simulink model "AGI_hydrogen"  (R2024b)
settings: Solver=VariableStepAuto  StartTime=0.0  StopTime=3  RelTol=1e-3
values from neighbouring files (symbols this model uses):
  ControlSampleTime = 1/8000    (= 0.000125)    [initTPHardware.m]
  HWSampleTime = ControlSampleTime/4    (= 3.125e-05)    [initTPHardware.m]
undefined symbols (not defined in the file or in its folder): DiscIntNeverNeededParam, fault_dur, Grid, Ion, LCL, Lithium, Manage, Param, SM, t_fault, Ts_Control, Ts_Power, V_DC, VSMCTRL
libraries: FriedrichLibrary x19, simulink x8, spsSeriesRLCBranchLib x7, spsThreePhaseSeriesRLCBranchLib x6, TriphaseHardwaremodule x6, powerlib_extras x6, spsThreePhaseVIMeasurementLib x5, spsVoltageMeasurementLib x5, spsThreePhaseBreakerLib x4, slpidlib x4, spsUniversalBridgeLib x3, spsCurrentMeasurementLib x3
(part 3 of 4)

== system AGI_hydrogen/Battery/VSM1/VSM/CONTROL/Virtual Circuit mit R und L ==
  Param : Inport
  Reset : Inport  Port=2
  i_dq0 : Inport  Port=3
  Phi : Inport  Port=4
  Bus Selector : BusSelector  OutputSignals=R1,L1
  Bus Selector1 : BusSelector  OutputSignals=R1t,tauR,L1t,tauL
  Current Predictor : Subsystem  Commented=on
  L_Matrix : Gain  Gain=[0 -1 0;1 0 0; 0 0 0]
  L_Matrix1 : Gain  Gain=[0 -1 0;1 0 0; 0 0 0]
  PT1 : Subsystem  mask{K=1, Init=0, Ts=ControlSampleTime}
      mask prompts: K "Gain"; Init "Initial input"; Ts "Sample time"
      mask DialogControl DescGroupVar Prompt: PT1 discrete
      mask DialogControl DescTextVar Prompt: Simple discrete PT1
      mask Display:
      | text(0.5,0.5,get_param(gcb,'K'),'HorizontalAlignment','center','VerticalAlignment','Bottom')
      | text(0.5,0.5,'1 + s.tau','HorizontalAlignment','center','VerticalAlignment','Top')
      | plot([0.3 0.7],[0.5 0.5])
  PT2 : Subsystem  mask{K=1, Init=0, Ts=ControlSampleTime}
      mask prompts: K "Gain"; Init "Initial input"; Ts "Sample time"
      mask DialogControl DescGroupVar Prompt: PT1 discrete
      mask DialogControl DescTextVar Prompt: Simple discrete PT1
      mask Display:
      | text(0.5,0.5,get_param(gcb,'K'),'HorizontalAlignment','center','VerticalAlignment','Bottom')
      | text(0.5,0.5,'1 + s.tau','HorizontalAlignment','center','VerticalAlignment','Top')
      | plot([0.3 0.7],[0.5 0.5])
  "Param " : InportShadow
  Phi1 : InportShadow  Port=4
  Product : Product  Multiplication=Matrix(*)
  Product1 : Product  Multiplication=Matrix(*)
  Product2 : Product  Multiplication=Matrix(*)
  R_Matrix : Gain  Gain=[1 0 0;0 1 0; 0 0 0]
  R_Matrix1 : Gain  Gain=[1 0 0;0 1 0; 0 0 0]
  Reset1 : InportShadow  Port=2
  Sum : Sum  Inputs=++|
  Sum1 : Sum  Inputs=++|
  Sum2 : Sum  Inputs=|++
  " u_dq0" : Outport
  wires:
  Param/1 -> Bus Selector/1
  Bus Selector/1 -> R_Matrix/1  "<R1>"
  i_dq0/1 -> Product/2, PT2/1(U), PT1/1(U)
  Bus Selector/2 -> L_Matrix/1  "<L1>"
  L_Matrix/1 -> Sum/1
  R_Matrix/1 -> Sum/2
  Sum/1 -> Product/1
  "Param "/1 -> Bus Selector1/1
  R_Matrix1/1 -> Product1/1
  Product1/1 -> Sum1/1
  Bus Selector1/1 -> R_Matrix1/1  "<R1t>"
  Bus Selector1/4 -> PT2/2(tau)  "<tauL>"
  Bus Selector1/2 -> PT1/2(tau)  "<tauR>"
  Bus Selector1/3 -> L_Matrix1/1  "<L1t>"
  L_Matrix1/1 -> Product2/1
  Product2/1 -> Sum1/2
  Sum2/1 -> " u_dq0"/1
  PT1/1(Y) -> Product1/2
  Phi/1 -> PT1/4(Phi)
  Phi1/1 -> PT2/4(Phi)
  Reset/1 -> PT1/3(Reset)
  Reset1/1 -> PT2/3(Reset)
  PT2/1(Y) -> Product2/2
  Product/1 -> Sum2/1

== system AGI_hydrogen/Battery/VSM1/VSM/CONTROL/Virtual Circuit1 ==
  Param : Inport
  Reset : Inport  Port=2
  i_dq0 : Inport  Port=3
  Phi : Inport  Port=4
  Bus Selector : BusSelector  OutputSignals=R1,L1
  Bus Selector1 : BusSelector  OutputSignals=R1t,tauR,L1t,tauL
  Current Predictor : Subsystem  Commented=on
  L_Matrix : Gain  Gain=[0 -1 0;1 0 0; 0 0 0]
  L_Matrix1 : Gain  Gain=[0 -1 0;1 0 0; 0 0 0]
  PT1 : Subsystem  mask{K=1, Init=0, Ts=ControlSampleTime}
      mask prompts: K "Gain"; Init "Initial input"; Ts "Sample time"
      mask DialogControl DescGroupVar Prompt: PT1 discrete
      mask DialogControl DescTextVar Prompt: Simple discrete PT1
      mask Display:
      | text(0.5,0.5,get_param(gcb,'K'),'HorizontalAlignment','center','VerticalAlignment','Bottom')
      | text(0.5,0.5,'1 + s.tau','HorizontalAlignment','center','VerticalAlignment','Top')
      | plot([0.3 0.7],[0.5 0.5])
  PT2 : Subsystem  Commented=on  mask{K=1, Init=0, Ts=ControlSampleTime}
      mask prompts: K "Gain"; Init "Initial input"; Ts "Sample time"
      mask DialogControl DescGroupVar Prompt: PT1 discrete
      mask DialogControl DescTextVar Prompt: Simple discrete PT1
      mask Display:
      | text(0.5,0.5,get_param(gcb,'K'),'HorizontalAlignment','center','VerticalAlignment','Bottom')
      | text(0.5,0.5,'1 + s.tau','HorizontalAlignment','center','VerticalAlignment','Top')
      | plot([0.3 0.7],[0.5 0.5])
  "Param " : InportShadow
  Phi1 : InportShadow  Port=4
  Product : Product  Multiplication=Matrix(*)
  Product1 : Product  Multiplication=Matrix(*)
  Product2 : Product  Commented=on  Multiplication=Matrix(*)
  Product3 : Product  Multiplication=Matrix(*)
  R_Matrix : Gain  Gain=[1 0 0;0 1 0; 0 0 0]
  R_Matrix1 : Gain  Gain=[1 0 0;0 1 0; 0 0 0]
  Reset1 : InportShadow  Port=2
  Scope : Scope  NumInputPorts=2
  Scope1 : Scope
  Sum : Sum  Inputs=++|
  Sum1 : Sum  Inputs=++|
  Sum2 : Sum  Inputs=|++
  " u_dq0" : Outport
  wires:
  Param/1 -> Bus Selector/1
  Bus Selector/1 -> R_Matrix/1  "<R1>"
  i_dq0/1 -> PT2/1(U), PT1/1(U), Product3/2, Product/2
  Bus Selector/2 -> L_Matrix/1  "<L1>"
  L_Matrix/1 -> Sum/1
  R_Matrix/1 -> Product3/1, Sum/2
  Sum/1 -> Product/1
  "Param "/1 -> Bus Selector1/1
  Product/1 -> Sum2/1
  R_Matrix1/1 -> Product1/1
  Product1/1 -> Scope/2, Sum1/1
  Bus Selector1/1 -> R_Matrix1/1  "<R1t>"
  Bus Selector1/4 -> PT2/2(tau)  "<tauL>"
  Bus Selector1/2 -> PT1/2(tau)  "<tauR>"
  Bus Selector1/3 -> L_Matrix1/1  "<L1t>"
  L_Matrix1/1 -> Product2/1
  PT2/1(Y) -> Product2/2
  Product2/1 -> Scope1/1, Sum1/2
  Sum1/1 -> Sum2/2
  Sum2/1 -> " u_dq0"/1
  PT1/1(Y) -> Product1/2
  Phi1/1 -> PT2/4(Phi)
  Reset/1 -> PT1/3(Reset)
  Reset1/1 -> PT2/3(Reset)
  Product3/1 -> Scope/1

== system AGI_hydrogen/Battery/VSM1/VSM/CONTROL/active_damping ==
  enable_damp_dq : Inport
  Reset : Inport  Port=2
  u_dq0 : Inport  Port=3
  Phi : Inport  Port=4
  Bus Selector : BusSelector  OutputSignals=Damp_dq,Damp_dq,Damp_CM,OmLead,OmLag
  Integrator (inertia) : DiscreteIntegrator  gainval=1  ExternalReset=rising  InitialConditionSource=external  InitialCondition=1  SampleTime=ControlSampleTime  ICPrevOutput=DiscIntNeverNeededParam  ICPrevScaledInput=DiscIntNeverNeededParam
  Mux : Mux  Inputs=3
  Product{,1..3} (4 alike) : Product
  Sum : Sum  Inputs=|+-
  Sum2 : Sum  Inputs=++|
  Unit Delay2 : UnitDelay  InitialCondition=[0 0 0]  SampleTime=ControlSampleTime  HasFrameUpgradeWarning=on
  dq0->ab0 phi : FriedrichLibrary/Transformations/dq0->ab0 phi  SystemSampleTime=-1  VariantActivationTime=update diagram  AllowFlexibleInterface=on  Latency=0  AutoFrameSizeCalculation=off
  damp_dq0 : Outport  VectorParamsAs1DForOutWhenUnconnected=off
  wires:
  Product2/1 -> Sum/1
  Integrator (inertia)/1 -> Unit Delay2/1, Sum2/2
  Product3/1 -> Sum/2
  Sum2/1 -> Product3/1, Product1/2
  Sum/1 -> Integrator (inertia)/1
  enable_damp_dq/1 -> Bus Selector/1
  Bus Selector/1 -> Mux/1  "<Damp_dq>"
  Bus Selector/2 -> Mux/2  "<Damp_dq>"
  Bus Selector/3 -> Mux/3  "<Damp_CM>"
  u_dq0/1 -> Product/2
  Product/1 -> Sum2/1, Product2/2
  Mux/1 -> Product1/1, Product/1  "enable"
  Product1/1 -> damp_dq0/1
  Phi/1 -> dq0->ab0 phi/2
  Reset/1 -> Integrator (inertia)/2
  Unit Delay2/1 -> dq0->ab0 phi/1
  dq0->ab0 phi/1 -> Integrator (inertia)/3
  Bus Selector/4 -> Product2/1  "<OmLead>"
  Bus Selector/5 -> Product3/2  "<OmLag>"

== system AGI_hydrogen/Battery/VSM1/VSM/CONTROL/dq0 to duty ==
  phi_rad : Inport
  u_dq0 : Inport  Port=2
  u_dc : Inport  Port=3
  Bias : Bias  Bias=Ctrl.PWM.tauT*Ctrl.PU.omegab  SaturateOnIntegerOverflow=off
  Bus Creator3 : BusCreator  Inputs=2
  Divide : Product  Inputs=*/
  Gain : Gain  Gain=eye(NrChannels,3)  Multiplication=Matrix(K*u)
  Modulation : FriedrichLibrary/Transformations/Modulation  Method=Sine Modulation  Ts=ControlSampleTime
  SMA : FriedrichLibrary/Discrete Stuff/SMA  n_samples=1/ControlSampleTime/100  init_out=0
  Saturation : Saturate  UpperLimit=inf  LowerLimit=1
  Signal Specification1 : SignalSpecification
  dq0->ab0 phi : FriedrichLibrary/Transformations/dq0->ab0 phi  SystemSampleTime=-1  VariantActivationTime=update diagram  AllowFlexibleInterface=on  Latency=0  AutoFrameSizeCalculation=off
  d : Outport  VectorParamsAs1DForOutWhenUnconnected=off
  pwmDiag : Outport  Port=2  VectorParamsAs1DForOutWhenUnconnected=off
  wires:
  phi_rad/1 -> Bus Creator3/2, Bias/1  "phi"
  u_dq0/1 -> dq0->ab0 phi/1
  Divide/1 -> Modulation/1  "ab0 norm"
  dq0->ab0 phi/1 -> Divide/1
  Modulation/1 -> Gain/1
  Bias/1 -> dq0->ab0 phi/2
  u_dc/1 -> Saturation/1
  Bus Creator3/1 -> pwmDiag/1  "pwmDiag"
  Gain/1 -> Bus Creator3/1, Signal Specification1/1  "pwm"
  Signal Specification1/1 -> d/1
  Saturation/1 -> SMA/1
  SMA/1 -> Divide/2

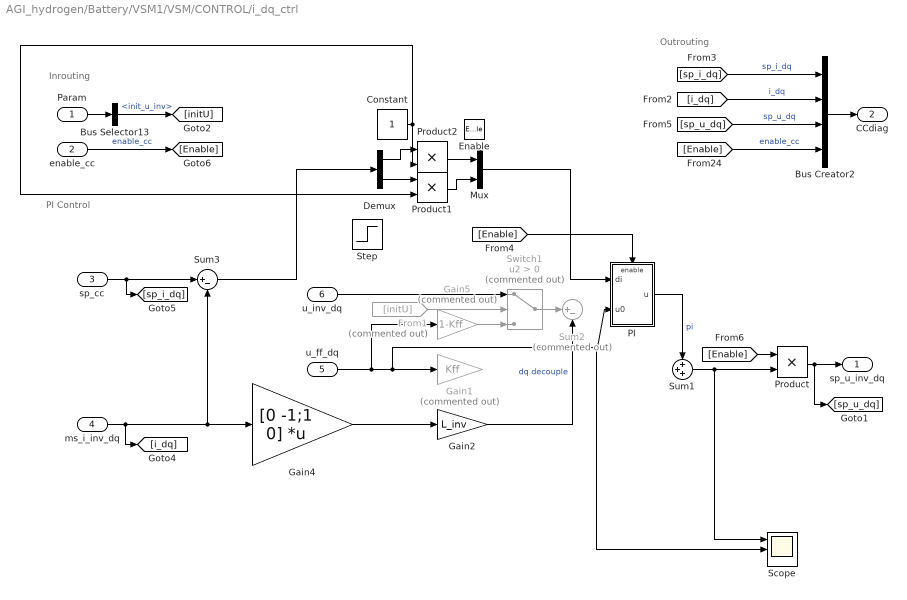
== system AGI_hydrogen/Battery/VSM1/VSM/CONTROL/i_dq_ctrl ==
  note: Inrouting
  note: Outrouting
  note: PI Control
  Param : Inport
  enable_cc : Inport  Port=2
  sp_cc : Inport  Port=3
  ms_i_inv_dq : Inport  Port=4
  u_ff_dq : Inport  Port=5
  u_inv_dq : Inport  Port=6
  Enable : EnablePort  StatesWhenEnabling=reset
  Bus Creator2 : BusCreator  Inputs=4
  Bus Selector13 : BusSelector  OutputSignals=init_u_inv
  Constant : Constant
  Demux : Demux  Outputs=2
  From1 : From  Commented=on  GotoTag=initU
  Gain1 : Gain  Commented=on  Gain=Kff
  Gain2 : Gain  Gain=L_inv
  Gain4 : Gain  Gain=[0 -1;1 0]  Multiplication=Matrix(K*u)
  Gain5 : Gain  Commented=on  Gain=1-Kff
  Mux : Mux  Inputs=2
  PI : Subsystem
  Product : Product
  Product1 : Product
  Product2 : Product
  Scope : Scope  NumInputPorts=3
  Step : Step  Time=8  Before=1  After=0  SampleTime=0
  Sum1 : Sum  Inputs=+++
  Sum2 : Sum  Commented=on  Inputs=|+-
  Sum3 : Sum  Inputs=|+-
  Switch1 : Switch  Commented=on  Criteria=u2 > Threshold  SaturateOnIntegerOverflow=off  InputSameDT=off
  sp_u_inv_dq : Outport  VectorParamsAs1DForOutWhenUnconnected=off
  CCdiag : Outport  Port=2  VectorParamsAs1DForOutWhenUnconnected=off
  wires:
  Switch1/1 -> Sum2/1
  Gain4/1 -> Gain2/1
  Gain2/1 -> Sum2/2  "dq decouple"
  From1/1 -> Switch1/2
  Sum1/1 -> Scope/1, Product/2
  u_inv_dq/1 -> Switch1/1
  [Enable] -> PI/Enable
  Sum3/1 -> Demux/1
  sp_cc/1 -> [sp_i_dq], Sum3/1
  Param/1 -> Bus Selector13/1
  Bus Selector13/1 -> [initU]  "<init_u_inv>"
  [Enable] -> Product/1
  [sp_u_dq] -> Bus Creator2/3  "sp_u_dq"
  enable_cc/1 -> [Enable]  "enable_cc"
  [Enable] -> Bus Creator2/4  "enable_cc"
  Bus Creator2/1 -> CCdiag/1
  [sp_i_dq] -> Bus Creator2/1  "sp_i_dq"
  [i_dq] -> Bus Creator2/2  "i_dq"
  u_ff_dq/1 -> Scope/2, PI/2(u0), Gain1/1, Gain5/1
  Gain5/1 -> Switch1/3
  Product/1 -> sp_u_inv_dq/1, [sp_u_dq]
  ms_i_inv_dq/1 -> [i_dq], Sum3/2, Gain4/1
  Mux/1 -> PI/1(di)
  Demux/2 -> Product1/1
  Product1/1 -> Mux/2
  Product2/1 -> Mux/1
  Demux/1 -> Product2/1
  Constant/1 -> Product2/2, Product1/2
  PI/1(u) -> Sum1/1  "pi"

== system AGI_hydrogen/Battery/VSM1/VSM/MANAGEMENT/Subsystem1 ==
  In1 : Inport
  <i_inv_dq0> : Inport  Port=2
  <u_cap_ab0> : Inport  Port=3
  <PQ_out> : Inport  Port=4
  enable : Inport  Port=5
  "AL brechen AL nicht mit FCN lösbar " : Memory
  Add2 : Sum  Inputs=+-
  Constant : Constant
  Divide : Product  Inputs=*/
  Math Function1 : Math  Operator=square  SignedPower=on
  Math Function2 : Math  Operator=square  SignedPower=on
  Selector2 : Selector  InputPortWidth=3  IndexOptions=Index vector (dialog)  Indices=[1 2]  OutputSizes=1
  Sqrt1 : Sqrt
  Sqrt2 : Sqrt
  Subsystem : Subsystem
  Subsystem1 : Subsystem
  Sum of Elements1 : Sum  Inputs=+
  Sum of Elements2 : Sum  Inputs=+
  CC : Outport
  sp_CC : Outport  Port=2
  wires:
  Sum of Elements1/1 -> Sqrt2/1
  Selector2/1 -> Math Function2/1
  Math Function1/1 -> Sum of Elements1/1
  Sqrt2/1 -> Subsystem/3(iabs), Subsystem1/2(In2)
  Sum of Elements2/1 -> Sqrt1/1
  "AL brechen AL nicht mit FCN lösbar "/1 -> Subsystem/1(i_inv)
  Sqrt1/1 -> Divide/2, Subsystem/4(U_cap)
  Math Function2/1 -> Sum of Elements2/1
  <u_cap_ab0>/1 -> Selector2/1
  <i_inv_dq0>/1 -> "AL brechen AL nicht mit FCN lösbar "/1
  Subsystem/1(i_sp) -> sp_CC/1  "sp_CC"
  In1/1 -> Math Function1/1
  Subsystem/2(CC) -> CC/1
  <PQ_out>/1 -> Divide/1, Subsystem/2(PQ_out)
  Subsystem1/1(i_pq_pre) -> Subsystem/5(PQ_pre)
  Divide/1 -> Subsystem1/1(In1)
  Constant/1 -> Add2/1
  enable/1 -> Add2/2, Subsystem/Enable
  Add2/1 -> Subsystem1/Enable
  Subsystem1/2(i_abs_pre) -> Subsystem/6(i abs_pre)

== system AGI_hydrogen/Battery/VSM1/VSM/MANAGEMENT/current_watchdog ==
  |i| set : Inport
  |i| reset : Inport  Port=2
  i_ab : Inport  Port=3
  sp_gain : Inport  Port=4
  PQ : Inport  Port=5
  i_inv : Inport  Port=6
  active_current_watchdog : EnablePort  StatesWhenEnabling=reset
  Divide : Product  Inputs=/**
  MATLAB Function : MATLAB Function  Commented=on  TreatAsAtomicUnit=on
  Math Function1 : Math  Operator=square  SignedPower=on
  Math Function2 : Math  Operator=square  SignedPower=on
  Math Function3 : Math  Operator=square  SignedPower=on
  Relational Operator : RelationalOperator  Operator=<=  OutDataTypeStr=boolean  InputSameDT=off
  Relational Operator1 : RelationalOperator  Operator=<=  OutDataTypeStr=boolean  InputSameDT=off
  S-R Flip-Flop1 : simulink_extras/Flip Flops/S-R Flip-Flop  initial_condition=0
  Scope : Scope  NumInputPorts=3
  Scope1 : Scope
  Sum of Elements1 : Sum  Inputs=+
  Terminator1 : Terminator
  enable_cc : Outport  VectorParamsAs1DForOutWhenUnconnected=off
  sp_gain_wd : Outport  Port=2  VectorParamsAs1DForOutWhenUnconnected=off
  wires:
  Math Function2/1 -> Relational Operator/1, MATLAB Function/2(set)
  i_ab/1 -> Math Function1/1
  Sum of Elements1/1 -> Relational Operator1/1, MATLAB Function/1(abs), Relational Operator/2
  Math Function1/1 -> Sum of Elements1/1
  Relational Operator1/1 -> S-R Flip-Flop1/2
  S-R Flip-Flop1/2 -> Terminator1/1
  Math Function3/1 -> Relational Operator1/2
  |i| reset/1 -> Divide/2, Math Function3/1
  |i| set/1 -> Divide/1, Math Function2/1
  sp_gain/1 -> Divide/3
  MATLAB Function/1(CC) -> enable_cc/1, Scope/1
  MATLAB Function/2(i) -> sp_gain_wd/1
  PQ/1 -> Scope1/1, MATLAB Function/3(p)
  i_inv/1 -> MATLAB Function/4(i_inv)

== system AGI_hydrogen/Battery/VSM1/VSM/MANAGEMENT/sp_VSM ==
  EnableRateLimit : Inport
  CMD : Inport  Port=2
  MEAS : Inport  Port=3
  Bus Creator : BusCreator  Inputs=3
  Bus Selector1 : BusSelector  OutputSignals=u_out.u_out_ab0
  Bus Selector6 : BusSelector  OutputSignals=Param.VSM.sp_f,Param.VSM.sp_E,Param.VSM.sp_PQ,Param.VSM.sp_PQ_limit
  "CMD " : InportShadow  Port=2
  E(PQ) : Subsystem
  PQ(U) Limit : Subsystem
  RateLimit : Subsystem
  Saturation : Saturate  UpperLimit=1  LowerLimit=-1
  sp_VSM : Outport  VectorParamsAs1DForOutWhenUnconnected=off
  wires:
  E(PQ)/1(sp_E) -> Bus Creator/2  "sp_E"
  Bus Selector6/2 -> E(PQ)/1(E)  "<sp_E>"
  Bus Selector6/3 -> Saturation/1  "<sp_PQ>"
  EnableRateLimit/1 -> RateLimit/Enable  "ENABLED"
  RateLimit/1(PQslow) -> E(PQ)/3(sp_PQ), PQ(U) Limit/1(sp_PQ)
  Bus Selector1/1 -> PQ(U) Limit/3(u_out)  "<u_out_ab0>"
  Bus Selector6/4 -> PQ(U) Limit/2(enable)  "<sp_PQ_limit>"
  PQ(U) Limit/1(sp_PQ_limit) -> Bus Creator/3  "sp_PQ"
  CMD/1 -> Bus Selector6/1
  MEAS/1 -> Bus Selector1/1
  Bus Selector6/1 -> Bus Creator/1  "<sp_f>"
  Bus Creator/1 -> sp_VSM/1
  "CMD "/1 -> E(PQ)/2(cmd)
  Saturation/1 -> RateLimit/1(PQ)

== system AGI_hydrogen/Battery/VSM1/VSM/Meas/SI -> pu ==
  MeasIn : Inport
  Bus Creator1 : BusCreator  Inputs=5
  Bus Selector : BusSelector  OutputSignals=meas_u_out,meas_i_out,meas_i_inverter,meas_u_dc,meas_u_cap
  Normalize : Gain  Gain=1/PU.Ub  OutDataTypeStr=double  RndMeth=Round
  Normalize1 : Gain  Gain=1/PU.Ib  OutDataTypeStr=double  RndMeth=Round
  Normalize2 : Gain  Gain=1/PU.Ib  OutDataTypeStr=double  RndMeth=Round
  Normalize3 : Gain  Gain=1/PU.Ub  OutDataTypeStr=double  RndMeth=Round
  Normalize4 : Gain  Gain=1/PU.Ub/2  OutDataTypeStr=double  RndMeth=Round
  MeasOut : Outport  VectorParamsAs1DForOutWhenUnconnected=off
  wires:
  Normalize3/1 -> Bus Creator1/5  "meas_u_cap"
  Bus Selector/5 -> Normalize3/1  "<meas_u_cap>"
  Bus Selector/4 -> Normalize4/1  "<meas_u_dc>"
  Bus Selector/3 -> Normalize1/1  "<meas_i_inverter>"
  Bus Selector/2 -> Normalize2/1  "<meas_i_out>"
  Bus Selector/1 -> Normalize/1  "<meas_u_out>"
  Bus Creator1/1 -> MeasOut/1
  Normalize4/1 -> Bus Creator1/4  "meas_vol_dc"
  Normalize2/1 -> Bus Creator1/2  "meas_i_out"
  Normalize1/1 -> Bus Creator1/3  "meas_i_inverter"
  Normalize/1 -> Bus Creator1/1  "meas_u_out"
  MeasIn/1 -> Bus Selector/1

== system AGI_hydrogen/Battery/VSM1/VSM/Meas/meas_i_inv ==
  abc : Inport
  phi : Inport  Port=2
  Bus Creator1 : BusCreator  Inputs=3
  PhN->ab2 : FriedrichLibrary/Transformations/PhN->ab0  SystemSampleTime=-1  VariantActivationTime=update diagram  AllowFlexibleInterface=on  Latency=0  AutoFrameSizeCalculation=off
  ab0->dq0-faster : FriedrichLibrary/Transformations/ab0->dq0-faster  SystemSampleTime=-1  VariantActivationTime=update diagram  AllowFlexibleInterface=on  Latency=0  AutoFrameSizeCalculation=off
  i_inv_x : Outport  VectorParamsAs1DForOutWhenUnconnected=off
  wires:
  ab0->dq0-faster/1 -> Bus Creator1/3  "i_inv_dq0"
  PhN->ab2/1 -> Bus Creator1/2, ab0->dq0-faster/1  "i_inv_ab0"
  abc/1 -> Bus Creator1/1, PhN->ab2/1  "i_inv_abc"
  phi/1 -> ab0->dq0-faster/2
  Bus Creator1/1 -> i_inv_x/1

== system AGI_hydrogen/Battery/VSM1/VSM/Meas/meas_i_out ==
  abc : Inport
  phi : Inport  Port=2
  Bus Creator1 : BusCreator  Inputs=3
  PhN->ab2 : FriedrichLibrary/Transformations/PhN->ab0  SystemSampleTime=-1  VariantActivationTime=update diagram  AllowFlexibleInterface=on  Latency=0  AutoFrameSizeCalculation=off
  ab0->dq0-faster : FriedrichLibrary/Transformations/ab0->dq0-faster  SystemSampleTime=-1  VariantActivationTime=update diagram  AllowFlexibleInterface=on  Latency=0  AutoFrameSizeCalculation=off
  i_out_x : Outport  VectorParamsAs1DForOutWhenUnconnected=off
  wires:
  ab0->dq0-faster/1 -> Bus Creator1/3  "i_out_dq0"
  PhN->ab2/1 -> Bus Creator1/2, ab0->dq0-faster/1  "i_out_ab0"
  abc/1 -> Bus Creator1/1, PhN->ab2/1  "i_out_abc"
  phi/1 -> ab0->dq0-faster/2
  Bus Creator1/1 -> i_out_x/1

== system AGI_hydrogen/Battery/VSM1/VSM/Meas/meas_u_cap ==
  abc : Inport
  phi : Inport  Port=2
  Bus Creator1 : BusCreator  Inputs=3
  PhN->ab2 : FriedrichLibrary/Transformations/PhN->ab0  SystemSampleTime=-1  VariantActivationTime=update diagram  AllowFlexibleInterface=on  Latency=0  AutoFrameSizeCalculation=off
  ab0->dq0-faster : FriedrichLibrary/Transformations/ab0->dq0-faster  SystemSampleTime=-1  VariantActivationTime=update diagram  AllowFlexibleInterface=on  Latency=0  AutoFrameSizeCalculation=off
  u_cap_x : Outport  VectorParamsAs1DForOutWhenUnconnected=off
  wires:
  Bus Creator1/1 -> u_cap_x/1
  phi/1 -> ab0->dq0-faster/2
  abc/1 -> PhN->ab2/1, Bus Creator1/1  "u_cap_abc"
  PhN->ab2/1 -> ab0->dq0-faster/1, Bus Creator1/2  "u_cap_ab0"
  ab0->dq0-faster/1 -> Bus Creator1/3  "u_cap_dq0"

== system AGI_hydrogen/Battery/VSM1/VSM/Meas/meas_u_out ==
  abc : Inport
  phi : Inport  Port=2
  Bus Creator1 : BusCreator  Inputs=3
  PhN->ab2 : FriedrichLibrary/Transformations/PhN->ab0  SystemSampleTime=-1  VariantActivationTime=update diagram  AllowFlexibleInterface=on  Latency=0  AutoFrameSizeCalculation=off
  ab0->dq0-faster : FriedrichLibrary/Transformations/ab0->dq0-faster  SystemSampleTime=-1  VariantActivationTime=update diagram  AllowFlexibleInterface=on  Latency=0  AutoFrameSizeCalculation=off
  u_out_x : Outport  VectorParamsAs1DForOutWhenUnconnected=off
  wires:
  Bus Creator1/1 -> u_out_x/1
  phi/1 -> ab0->dq0-faster/2
  abc/1 -> PhN->ab2/1, Bus Creator1/1  "u_out_abc"
  PhN->ab2/1 -> ab0->dq0-faster/1, Bus Creator1/2  "u_out_ab0"
  ab0->dq0-faster/1 -> Bus Creator1/3  "u_out_dq0"

== system AGI_hydrogen/Battery/VSM1/command_center/cmd_VSM/Current Control ==
  note: else: init with u cap
  Bus Creator6 : BusCreator  Inputs=5
  Bus Creator7 : BusCreator  Inputs=3
  Init with u_inv [0/1] : Constant  Value=VSMCTRL.CC.init_uinv
  activate : Constant  Value=VSMCTRL.CC.activate
  external_stop_cc1 : Constant  Value=0
  external_stop_cc4 : Constant  Value=0
  i_reset_abs : Constant  Value=VSMCTRL.CC.i_reset
  i_set_abs : Constant  Value=VSMCTRL.CC.i_set
  i_sp_gain : Constant  Value=VSMCTRL.CC.i_sp_gain
  Current Control : Outport  VectorParamsAs1DForOutWhenUnconnected=off
  wires:
  activate/1 -> Bus Creator7/1  "activate"
  i_reset_abs/1 -> Bus Creator7/3  "abs_i_reset"
  Bus Creator7/1 -> Bus Creator6/5  "watchdog"
  external_stop_cc4/1 -> Bus Creator6/2  "ex_start_cc"
  i_set_abs/1 -> Bus Creator7/2  "abs_i_set"
  i_sp_gain/1 -> Bus Creator6/4  "i_sp_gain"
  external_stop_cc1/1 -> Bus Creator6/3  "ex_stop_cc"
  Init with u_inv [0/1]/1 -> Bus Creator6/1  "init_u_inv"
  Bus Creator6/1 -> Current Control/1  "CC"

== system AGI_hydrogen/Battery/VSM1/command_center/cmd_VSM/Damping ==
  Bus Creator5 : BusCreator  Inputs=4
  EnableDamp_CM [0/1] : Constant  Value=VSMCTRL.VTFF.EnableCM
  EnableDamp_dq [0/1] : Constant  Value=VSMCTRL.VTFF.EnableDQ
  Omega Lag : Constant  Value=VSMCTRL.VTFF.OmLag
  Omega Lead : Constant  Value=VSMCTRL.VTFF.OmLead
  Damping : Outport  VectorParamsAs1DForOutWhenUnconnected=off
  wires:
  EnableDamp_CM [0/1]/1 -> Bus Creator5/2  "Damp_CM"
  EnableDamp_dq [0/1]/1 -> Bus Creator5/1  "Damp_dq"
  Bus Creator5/1 -> Damping/1
  Omega Lead/1 -> Bus Creator5/3  "OmLead"
  Omega Lag/1 -> Bus Creator5/4  "OmLag"

== system AGI_hydrogen/Battery/VSM1/command_center/cmd_VSM/Manage ==
  Bus Creator : BusCreator  Inputs=2
  connect : Constant
  enable : Constant
  Manage : Outport  VectorParamsAs1DForOutWhenUnconnected=off
  wires:
  Bus Creator/1 -> Manage/1
  connect/1 -> Bus Creator/1  "connect"
  enable/1 -> Bus Creator/2  "enable"

== system AGI_hydrogen/Battery/VSM1/command_center/cmd_VSM/Virtual Circuit ==
  Bus Creator9 : BusCreator  Inputs=7
  Virtual L1 : Constant  Value=VSMCTRL.VC.L1
  Virtual L1t : Constant  Value=VSMCTRL.VC.L1t
  Virtual R1 : Constant  Value=VSMCTRL.VC.R1
  Virtual R1t : Constant  Value=VSMCTRL.VC.R1t
  tau HP Slow : Constant  Value=VSMCTRL.VC.tauSlow
  tau Virtual L1 : Constant  Value=VSMCTRL.VC.tauL
  tau Virtual R1 : Constant  Value=VSMCTRL.VC.tauR
  Virtual Circuit : Outport  VectorParamsAs1DForOutWhenUnconnected=off
  wires:
  Virtual R1/1 -> Bus Creator9/1  "R1"
  Virtual R1t/1 -> Bus Creator9/2  "R1t"
  Virtual L1t/1 -> Bus Creator9/4  "L1t"
  Bus Creator9/1 -> Virtual Circuit/1
  Virtual L1/1 -> Bus Creator9/3  "L1"
  tau Virtual R1/1 -> Bus Creator9/5  "tauR"
  tau Virtual L1/1 -> Bus Creator9/6  "tauL"
  tau HP Slow/1 -> Bus Creator9/7  "tauS"

== system AGI_hydrogen/Battery/VSM1/command_center/cmd_VSM/Virtual Synchronous Machine ==
  note: 0 Dekaktiviert Init Tiefpass
  note: 0 Dekaktiviert Init Tiefpass
  Bus Creator3 : BusCreator  Inputs=12
  E(sp_PQ) : Constant  Value=VSMCTRL.SP.E_comp
  Ta : Constant  Value=VSMCTRL.VSM.Ta
  Ta1 : Constant  Value=VSMCTRL.VSM.kpf
  Ta2 : Constant  Value=VSMCTRL.VSM.kdf
  Ta3 : Constant  Value=VSMCTRL.VSM.ku
  Ta4 : Constant  Value=VSMCTRL.VSM.Tu
  Ta5 : Constant  Value=0
  Ta6 : Constant  Value=0
  sp_E [pu] : Constant  Value=VSMCTRL.SP.E
  sp_PQ [pu] : Constant  Value=VSMCTRL.SP.PQ
  sp_PQ(U) limit : Constant  Value=VSMCTRL.SP.PQU_lim
  sp_f [Hz] : Constant  Value=VSMCTRL.SP.f
  Virtual Synchronous Machine : Outport  VectorParamsAs1DForOutWhenUnconnected=off
  wires:
  sp_E [pu]/1 -> Bus Creator3/10  "sp_E"
  sp_PQ [pu]/1 -> Bus Creator3/9  "sp_PQ"
  sp_f [Hz]/1 -> Bus Creator3/8  "sp_f"
  sp_PQ(U) limit/1 -> Bus Creator3/11  "sp_PQ_limit"
  Ta/1 -> Bus Creator3/1  "Ta"
  Bus Creator3/1 -> Virtual Synchronous Machine/1
  Ta4/1 -> Bus Creator3/5  "Tu"
  Ta3/1 -> Bus Creator3/4  "ku"
  Ta2/1 -> Bus Creator3/3  "kdf"
  Ta1/1 -> Bus Creator3/2  "kpf"
  Ta6/1 -> Bus Creator3/7  "TPinit"
  Ta5/1 -> Bus Creator3/6  "Tuinit"
  E(sp_PQ)/1 -> Bus Creator3/12  "sp_E_comp"

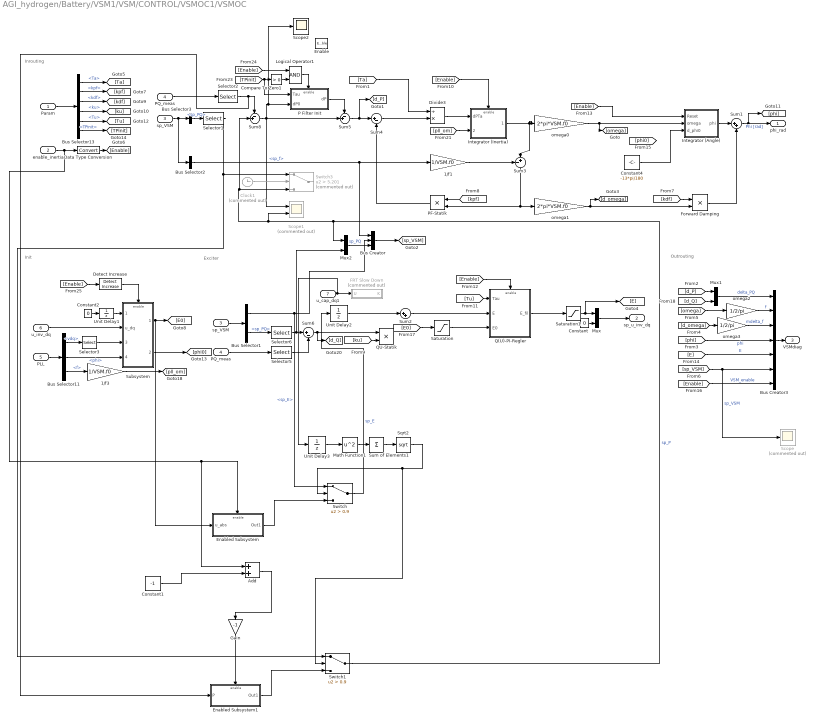
== system AGI_hydrogen/Battery/VSM1/VSM/CONTROL/VSMOC1/VSMOC ==
  note: Inrouting
  note: Exciter
  note: Init
  note: Outrouting
  Param : Inport
  enable_inertia : Inport  Port=2
  sp_VSM : Inport  Port=3
  PQ_meas : Inport  Port=4
  PLL : Inport  Port=5
  u_inv_dq : Inport  Port=6
  u_cap_dq1 : Inport  Port=7
  Enable : EnablePort  StatesWhenEnabling=reset
  1/f1 : Gain  Gain=1/VSM.f0
  1/f3 : Gain  Gain=1/VSM.f0
  Add : Sum
  Bus Creator : BusCreator  Inputs=3
  Bus Creator3 : BusCreator  Inputs=7
  Bus Selector1 : BusSelector  OutputSignals=sp_E,sp_PQ
  Bus Selector11 : BusSelector  OutputSignals=vdq,phi,f
  Bus Selector13 : BusSelector  OutputSignals=Ta,kpf,kdf,ku,Tu,TPinit
  Bus Selector2 : BusSelector  OutputSignals=sp_f
  Bus Selector3 : BusSelector  OutputSignals=sp_PQ
  Clock1 : Clock  Commented=on
  Compare To Zero1 : simulink/Logic and Bit Operations/Compare To Zero  relop=>  OutDataTypeStr=boolean
  Constant : Constant  Value=0
  Constant1 : Constant  Value=-1
  Constant2 : Constant  Value=0  SampleTime=ControlSampleTime
  Constant4 : Constant  Value=-13*pi/180
  Data Type Conversion : DataTypeConversion  SaturateOnIntegerOverflow=off  RndMeth=Floor
  Detect Increase : simulink/Logic and Bit Operations/Detect Increase  vinit=0.0  OutDataTypeStr=boolean
  Divide3 : Product  Inputs=/*
  Enabled Subsystem : Subsystem  TreatAsAtomicUnit=on
  Enabled Subsystem1 : Subsystem  TreatAsAtomicUnit=on
  FRT Slow Down : Subsystem  Commented=on
  Forward Damping : Product  Inputs=**
  Gain : Gain  Gain=-1
  Integrator (Angle) : Subsystem
  Integrator (Inertia) : Subsystem
  Logical Operator1 : Logic  AllPortsSameDT=off  OutDataTypeStr=boolean
  Math Function1 : Math  Operator=square  SignedPower=on
  Mux : Mux  Inputs=2
  Mux1 : Mux  Inputs=2
  Mux2 : Mux  Inputs=2
  P Filter Init : Subsystem
  PF-Statik : Product  Inputs=**
  "PQ_meas " : InportShadow  Port=4
  Q(U)-PI-Regler : Subsystem
  QU-Statik : Product  Inputs=**
  Saturation : Saturate  UpperLimit=1.8  LowerLimit=0.8*0
  Saturation1 : Saturate  UpperLimit=2
  Scope : Scope  Commented=on
  Scope1 : Scope  Commented=on  NumInputPorts=2
  Scope2 : Scope
  Selector1 : Selector  InputPortWidth=2  IndexOptions=Index vector (dialog)  Indices=1  OutputSizes=1
  Selector2 : Selector  InputPortWidth=2  IndexOptions=Index vector (dialog)  Indices=1  OutputSizes=1
  Selector3 : Selector  InputPortWidth=3  IndexOptions=Index vector (dialog)  Indices=[1 2]  OutputSizes=1
  Selector5 : Selector  InputPortWidth=2  IndexOptions=Index vector (dialog)  Indices=2  OutputSizes=1
  Selector6 : Selector  InputPortWidth=2  IndexOptions=Index vector (dialog)  Indices=2  OutputSizes=1
  Sqrt2 : Sqrt
  Subsystem : Subsystem
  Sum of Elements1 : Sum  Inputs=+
  Sum1 : Sum  Inputs=|++
  Sum2 : Sum  Inputs=|++
  Sum3 : Sum  Inputs=-+|
  Sum4 : Sum  Inputs=|+-
  Sum5 : Sum  Inputs=-+|
  Sum6 : Sum  Inputs=|+-
  Sum8 : Sum  Inputs=-+|
  Switch : Switch  Criteria=u2 > Threshold  Threshold=0.9  SaturateOnIntegerOverflow=off  InputSameDT=off
  Switch1 : Switch  Criteria=u2 > Threshold  Threshold=0.9  SaturateOnIntegerOverflow=off  InputSameDT=off
  Switch3 : Switch  Commented=on  Criteria=u2 > Threshold  Threshold=5.201  SaturateOnIntegerOverflow=off  InputSameDT=off
  Unit Delay1 : UnitDelay  InitialCondition=1  SampleTime=ControlSampleTime  HasFrameUpgradeWarning=on
  Unit Delay2 : UnitDelay  SampleTime=-1  HasFrameUpgradeWarning=on
  Unit Delay3 : UnitDelay  SampleTime=-1  HasFrameUpgradeWarning=on
  omega0 : Gain  Gain=2*pi*VSM.f0
  omega1 : Gain  Gain=2*pi*VSM.f0
  omega2 : Gain  Gain=1/2/pi
  omega3 : Gain  Gain=1/2/pi
  "sp_VSM " : InportShadow  Port=3
  phi_rad : Outport  VectorParamsAs1DForOutWhenUnconnected=off
  sp_u_inv_dq : Outport  Port=2  InitialOutput=[1 0]  VectorParamsAs1DForOutWhenUnconnected=off
  VSMdiag : Outport  Port=3  VectorParamsAs1DForOutWhenUnconnected=off
  wires:
  [Enable] -> Q(U)-PI-Regler/Enable
  Bus Selector11/2 -> Subsystem/4(phi_pll)  "<phi>"
  Selector5/1 -> Sum6/2
  Selector6/1 -> Mux2/2, Sum6/1
  1/f1/1 -> Sum3/1
  [d_Q] -> Mux1/2
  [d_P] -> Mux1/1
  Mux1/1 -> Bus Creator3/1  "delta_PQ"
  Selector2/1 -> Enabled Subsystem1/1(P), Sum8/1
  Sum6/1 -> QU-Statik/1, [d_Q]
  "sp_VSM "/1 -> Bus Selector1/1
  Bus Selector1/2 -> Selector6/1  "<sp_PQ>"
  "PQ_meas "/1 -> Selector5/1
  [kpf] -> PF-Statik/1
  [kdf] -> Forward Damping/1
  1/f3/1 -> [pll_om]
  Bus Selector11/3 -> 1/f3/1  "<f>"
  Integrator (Angle)/1(phi) -> Sum1/1
  Selector3/1 -> Subsystem/3(u_dq_pll)
  [Enable] -> Bus Creator3/7  "VSM_enable"
  Sum1/1 -> [phi], phi_rad/1  "Phi [rad]"
  Sum4/1 -> Divide3/2
  Sum3/1 -> PF-Statik/2, omega1/1
  Bus Selector2/1 -> Bus Creator/1, 1/f1/1  "<sp_f>"
  PLL/1 -> Bus Selector11/1
  Bus Creator3/1 -> VSMdiag/1
  [omega] -> omega2/1
  omega1/1 -> Forward Damping/2, [d_omega]
  [d_omega] -> omega3/1
  omega2/1 -> Bus Creator3/2  "f"
  omega3/1 -> Bus Creator3/3  "mdelta_f"
  [sp_VSM] -> Scope/1, Bus Creator3/6  "sp_VSM"
  PQ_meas/1 -> Selector2/1
  Bus Selector11/1 -> Selector3/1  "<vdq>"
  Divide3/1 -> Integrator (Inertia)/1(dPTa)
  [pll_om] -> Integrator (Inertia)/2(omega0 [pu])
  Mux/1 -> sp_u_inv_dq/1
  Constant/1 -> Mux/2
  Subsystem/2(u_ang) -> [phi0]
  Detect Increase/1 -> Subsystem/Enable
  Sum5/1 -> Sum4/1, [d_P]
  [TPinit] -> P Filter Init/1(Tau), Compare To Zero1/1
  Compare To Zero1/1 -> Logical Operator1/2
  Logical Operator1/1 -> P Filter Init/Enable
  [Enable] -> Logical Operator1/1
  Bus Selector13/5 -> [Tu]  "<Tu>"
  Bus Selector13/4 -> [ku]  "<ku>"
  Bus Selector13/3 -> [kdf]  "<kdf>"
  Bus Selector13/2 -> [kpf]  "<kpf>"
  Bus Selector13/1 -> [Ta]  "<Ta>"
  Param/1 -> Bus Selector13/1
  [Enable] -> Detect Increase/1
  u_inv_dq/1 -> Subsystem/2(u_dq)
  Constant2/1 -> Unit Delay1/1
  Unit Delay1/1 -> Subsystem/1(first_run)
  Data Type Conversion/1 -> [Enable]
  Sum2/1 -> Q(U)-PI-Regler/2(E)
  [ku] -> QU-Statik/2
  [E] -> Bus Creator3/5  "E"
  Bus Selector13/6 -> [TPinit]  "<TPinit>"
  [phi] -> Bus Creator3/4  "phi"
  [Tu] -> Q(U)-PI-Regler/1(Tau)
  Unit Delay2/1 -> Sum2/1
  [E0] -> Saturation/1
  [Enable] -> Integrator (Angle)/1(Reset)
  omega0/1 -> Integrator (Angle)/2(omega), [omega]
  Saturation1/1 -> [E], Mux/1
  Forward Damping/1 -> Sum1/2
  [Enable] -> Integrator (Inertia)/Enable
  Integrator (Inertia)/1(omega [pu]) -> omega0/1, Sum3/2
  Bus Selector3/1 -> Selector1/1  "<sp_PQ>"
  sp_VSM/1 -> Bus Selector2/1, Bus Selector3/1
  Sum8/1 -> Scope1/1, Sum5/2, Scope2/1, P Filter Init/2(dP0)
  [Ta] -> Divide3/1
  P Filter Init/1(dP) -> Sum5/1
  PF-Statik/1 -> Sum4/2
  Sqrt2/1 -> Switch1/2, Switch/2
  u_cap_dq1/1 -> Unit Delay3/1, FRT Slow Down/1(U)
  Sum of Elements1/1 -> Sqrt2/1
  Unit Delay3/1 -> Math Function1/1
  Math Function1/1 -> Sum of Elements1/1
  Bus Selector1/1 -> Bus Creator/2, Switch/1  "<sp_E>"
  enable_inertia/1 -> Add/1, Enabled Subsystem/Enable, Data Type Conversion/1
  Enabled Subsystem/1(Out1) -> Switch/3
  Subsystem/1(u_abs) -> Enabled Subsystem/1(u_abs), [E0]
  Enabled Subsystem1/1(Out1) -> Switch1/3
  Switch/1 -> Unit Delay2/1  "sp_E"
  Switch1/1 -> Scope1/2, Sum8/2, Switch3/3, Mux2/1  "sp_P"
  Clock1/1 -> Switch3/2
  Q(U)-PI-Regler/1(E_fil) -> Saturation1/1
  Selector1/1 -> Switch3/1, Switch1/1
  Constant1/1 -> Add/2
  Gain/1 -> Enabled Subsystem1/Enable
  Add/1 -> Gain/1
  Mux2/1 -> Bus Creator/3  "sp_PQ"
  Bus Creator/1 -> [sp_VSM]
  Constant4/1 -> Integrator (Angle)/3(d_phi0)
  Saturation/1 -> Q(U)-PI-Regler/3(E0)

== system AGI_hydrogen/Battery/VSM1/VSM/CONTROL/Virtual Circuit mit R und L/Current Predictor ==
  u : Inport
  Delay : Delay  DelayLength=1  InitialCondition=0
  Sum : Sum  Inputs=|-+
  Sum1 : Sum  Inputs=|++
  y : Outport
  wires:
  u/1 -> Sum/2, Sum1/2, Delay/1
  Delay/1 -> Sum/1
  Sum/1 -> Sum1/1
  Sum1/1 -> y/1

== system AGI_hydrogen/Battery/VSM1/VSM/CONTROL/Virtual Circuit mit R und L/PT1 ==
  U : Inport  SampleTime=Ts
  tau : Inport  Port=2  SampleTime=Ts
  Reset : Inport  Port=3  SampleTime=Ts
  Phi : Inport  Port=4
  Delay : Delay  DelayLength=1  InitialConditionSource=Input port  ExternalReset=Rising
      settings: InputPortMap=u0,r5,p4
  Divide : Product  Inputs=*/
  Gain : Gain  Gain=Ts
  Gain1 : Gain  Gain=K
  Saturation : Saturate  UpperLimit=inf  LowerLimit=Ts
  Sum : Sum  Inputs=|++
  Sum2 : Sum  Inputs=|+-
  Unit Delay2 : UnitDelay  InitialCondition=[0 0 0]  SampleTime=ControlSampleTime  HasFrameUpgradeWarning=on
  dq0->ab0 phi : FriedrichLibrary/Transformations/dq0->ab0 phi  SystemSampleTime=-1  VariantActivationTime=update diagram  Latency=0  AutoFrameSizeCalculation=off
  Y : Outport
  wires:
  Phi/1 -> dq0->ab0 phi/2
  Unit Delay2/1 -> dq0->ab0 phi/1
  Sum/1 -> Gain1/1, Unit Delay2/1, Delay/1
  Reset/1 -> Delay/2
  Saturation/1 -> Divide/2
  Divide/1 -> Sum/1
  tau/1 -> Saturation/1
  Delay/1 -> Sum2/2, Sum/2
  Gain/1 -> Divide/1
  U/1 -> Sum2/1
  Sum2/1 -> Gain/1
  Gain1/1 -> Y/1
  dq0->ab0 phi/1 -> Delay/3

== system AGI_hydrogen/Battery/VSM1/VSM/CONTROL/Virtual Circuit mit R und L/PT2 ==
  U : Inport  SampleTime=Ts
  tau : Inport  Port=2  SampleTime=Ts
  Reset : Inport  Port=3  SampleTime=Ts
  Phi : Inport  Port=4
  Delay : Delay  DelayLength=1  InitialConditionSource=Input port  ExternalReset=Rising
      settings: InputPortMap=u0,r5,p4
  Divide : Product  Inputs=*/
  Gain : Gain  Gain=Ts
  Gain1 : Gain  Gain=K
  Saturation : Saturate  UpperLimit=inf  LowerLimit=Ts
  Sum : Sum  Inputs=|++
  Sum2 : Sum  Inputs=|+-
  Unit Delay2 : UnitDelay  InitialCondition=[0 0 0]  SampleTime=ControlSampleTime  HasFrameUpgradeWarning=on
  dq0->ab0 phi1 : FriedrichLibrary/Transformations/dq0->ab0 phi  SystemSampleTime=-1  VariantActivationTime=update diagram  Latency=0  AutoFrameSizeCalculation=off
  Y : Outport
  wires:
  dq0->ab0 phi1/1 -> Delay/3
  Gain1/1 -> Y/1
  Sum2/1 -> Gain/1
  U/1 -> Sum2/1
  Gain/1 -> Divide/1
  Delay/1 -> Sum/2, Sum2/2
  tau/1 -> Saturation/1
  Divide/1 -> Sum/1
  Saturation/1 -> Divide/2
  Reset/1 -> Delay/2
  Sum/1 -> Delay/1, Unit Delay2/1, Gain1/1
  Unit Delay2/1 -> dq0->ab0 phi1/1
  Phi/1 -> dq0->ab0 phi1/2

== system AGI_hydrogen/Battery/VSM1/VSM/CONTROL/Virtual Circuit1/Current Predictor ==
  u : Inport
  Delay : Delay  DelayLength=1  InitialCondition=0
  Sum : Sum  Inputs=|-+
  Sum1 : Sum  Inputs=|++
  y : Outport
  wires:
  u/1 -> Sum/2, Sum1/2, Delay/1
  Delay/1 -> Sum/1
  Sum/1 -> Sum1/1
  Sum1/1 -> y/1

== system AGI_hydrogen/Battery/VSM1/VSM/CONTROL/Virtual Circuit1/PT1 ==
  U : Inport  SampleTime=Ts
  tau : Inport  Port=2  SampleTime=Ts
  Reset : Inport  Port=3  SampleTime=Ts
  Delay : Delay  DelayLength=1
  Divide : Product  Inputs=*/
  Gain : Gain  Gain=Ts
  Gain1 : Gain  Gain=K
  Saturation : Saturate  UpperLimit=inf  LowerLimit=Ts
  Sum : Sum  Inputs=|++
  Sum2 : Sum  Inputs=|+-
  Switch : Switch  Criteria=u2 > Threshold  SaturateOnIntegerOverflow=off  InputSameDT=off
  Y : Outport
  wires:
  Reset/1 -> Switch/2
  Saturation/1 -> Divide/2
  Divide/1 -> Sum/1
  tau/1 -> Saturation/1
  Delay/1 -> Sum2/2, Sum/2
  Gain/1 -> Divide/1
  U/1 -> Switch/1, Sum2/1
  Sum2/1 -> Gain/1
  Gain1/1 -> Y/1
  Switch/1 -> Gain1/1, Delay/1
  Sum/1 -> Switch/3

== system AGI_hydrogen/Battery/VSM1/VSM/CONTROL/Virtual Circuit1/PT2 ==
  U : Inport  SampleTime=Ts
  tau : Inport  Port=2  SampleTime=Ts
  Reset : Inport  Port=3  SampleTime=Ts
  Phi : Inport  Port=4
  Delay : Delay  DelayLength=1  InitialConditionSource=Input port  ExternalReset=Rising
      settings: InputPortMap=u0,r5,p4
  Divide : Product  Inputs=*/
  Gain : Gain  Gain=Ts
  Gain1 : Gain  Gain=K
  Saturation : Saturate  UpperLimit=inf  LowerLimit=Ts
  Sum : Sum  Inputs=|++
  Sum2 : Sum  Inputs=|+-
  Unit Delay2 : UnitDelay  InitialCondition=[0 0 0]  SampleTime=ControlSampleTime  HasFrameUpgradeWarning=on
  dq0->ab0 phi1 : FriedrichLibrary/Transformations/dq0->ab0 phi  SystemSampleTime=-1  VariantActivationTime=update diagram  Latency=0  AutoFrameSizeCalculation=off
  Y : Outport
  wires:
  dq0->ab0 phi1/1 -> Delay/3
  Gain1/1 -> Y/1
  Sum2/1 -> Gain/1
  U/1 -> Sum2/1
  Gain/1 -> Divide/1
  Delay/1 -> Sum/2, Sum2/2
  tau/1 -> Saturation/1
  Divide/1 -> Sum/1
  Saturation/1 -> Divide/2
  Reset/1 -> Delay/2
  Sum/1 -> Delay/1, Unit Delay2/1, Gain1/1
  Unit Delay2/1 -> dq0->ab0 phi1/1
  Phi/1 -> dq0->ab0 phi1/2

== system AGI_hydrogen/Battery/VSM1/VSM/CONTROL/i_dq_ctrl/PI ==
  di : Inport
  u0 : Inport  Port=2
  Enable : EnablePort  StatesWhenEnabling=reset
  Gain4 : Gain  Gain=Ki
  Gain5 : Gain  Gain=Kp
  Integrator (inertia) : DiscreteIntegrator  gainval=1  InitialConditionSource=external  InitialCondition=1  SampleTime=ControlSampleTime  ICPrevOutput=DiscIntNeverNeededParam  ICPrevScaledInput=DiscIntNeverNeededParam
  Product : Product
  Product1 : Product
  Step : Step  Time=8  Before=1  SampleTime=0
  Step1 : Step  Time=8.05+10  Before=1  After=0.1  SampleTime=0
  Sum2 : Sum  Inputs=++|
  u : Outport  VectorParamsAs1DForOutWhenUnconnected=off
  wires:
  u0/1 -> Integrator (inertia)/2
  Sum2/1 -> u/1
  di/1 -> Gain4/1, Gain5/1
  Integrator (inertia)/1 -> Sum2/2
  Gain5/1 -> Product/2
  Gain4/1 -> Product1/2
  Product1/1 -> Integrator (inertia)/1
  Product/1 -> Sum2/1
  Step/1 -> Product/1
  Step1/1 -> Product1/1

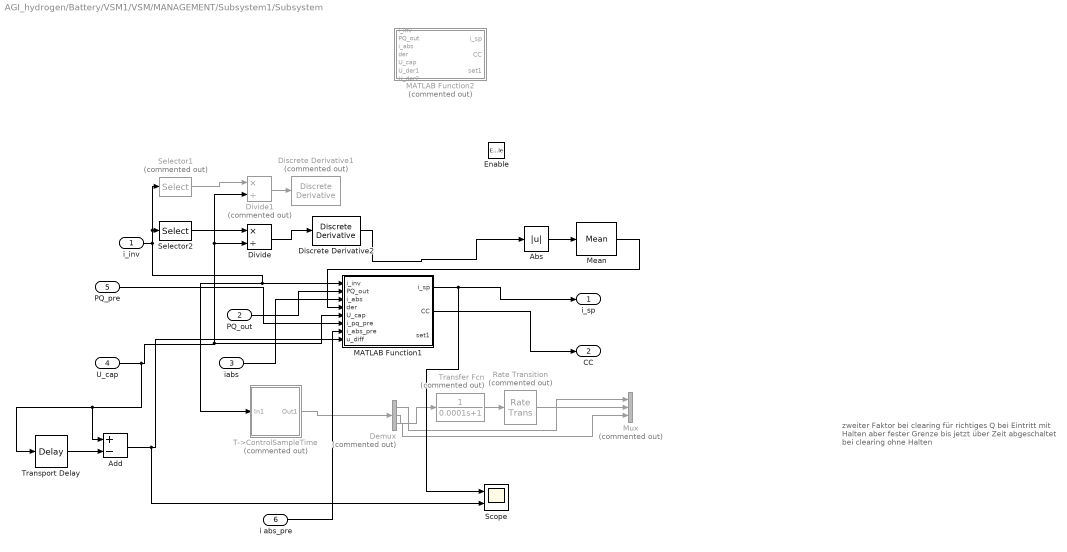
== system AGI_hydrogen/Battery/VSM1/VSM/MANAGEMENT/Subsystem1/Subsystem ==
  note: zweiter Faktor bei clearing für richtiges Q
      |
      | bei Eintritt mit Halten aber fester Grenze
      |
      | bis jetzt über Zeit abgeschaltet bei clearing ohne Halten
  i_inv : Inport
  PQ_out : Inport  Port=2
  iabs : Inport  Port=3
  U_cap : Inport  Port=4
  PQ_pre : Inport  Port=5
  i abs_pre : Inport  Port=6
  Enable : EnablePort
  Abs : Abs  SaturateOnIntegerOverflow=off
  Add : Sum  Inputs=+-
  Demux : Demux  Commented=on  Outputs=3
  Discrete Derivative1 : simulink/Discrete/Discrete Derivative  Commented=on  gainval=1.0  ICPrevScaledInput=0.0  OutMin=[]  OutMax=[]  OutDataType=fixdt(1, 16)  OutScaling=2^-10  DoSatur=off
  Discrete Derivative2 : simulink/Discrete/Discrete Derivative  gainval=1.0  ICPrevScaledInput=0.0  OutMin=[]  OutMax=[]  OutDataType=fixdt(1, 16)  OutScaling=2^-10  DoSatur=off
  Divide : Product  Inputs=*/
  Divide1 : Product  Commented=on  Inputs=*/
  MATLAB Function1 : MATLAB Function  TreatAsAtomicUnit=on  SystemSampleTime=ControlSampleTime
  MATLAB Function2 : MATLAB Function  Commented=on  TreatAsAtomicUnit=on  SystemSampleTime=ControlSampleTime
  Mean : spsMeanLib/Mean  Freq=2000/2  Vinit=0  Ts=0
  Mux : Mux  Commented=on  Inputs=3
  Rate Transition : RateTransition  Commented=on  OutPortSampleTime=ControlSampleTime
  Scope : Scope  NumInputPorts=2
  Selector1 : Selector  Commented=on  InputPortWidth=3  IndexOptions=Index vector (dialog)  Indices=2  OutputSizes=1
  Selector2 : Selector  InputPortWidth=3  IndexOptions=Index vector (dialog)  Indices=1  OutputSizes=1
  T->ControlSampleTime : Subsystem  Commented=on  TreatAsAtomicUnit=on  SystemSampleTime=ControlSampleTime
  Transfer Fcn : TransferFcn  Commented=on  Denominator=[0.0001 1]
  Transport Delay : TransportDelay  DelayTime=0.002
  i_sp : Outport
  CC : Outport  Port=2
  wires:
  PQ_out/1 -> MATLAB Function1/2(PQ_out)
  iabs/1 -> MATLAB Function1/3(i_abs)
  T->ControlSampleTime/1(Out1) -> Demux/1
  U_cap/1 -> Add/1, Transport Delay/1, Divide1/2, Divide/2, MATLAB Function1/5(U_cap)
  Demux/2 -> Transfer Fcn/1
  Transfer Fcn/1 -> Rate Transition/1
  Demux/1 -> Mux/1
  Demux/3 -> Mux/3
  Rate Transition/1 -> Mux/2
  MATLAB Function1/1(i_sp) -> Scope/1, i_sp/1
  MATLAB Function1/2(CC) -> CC/1
  Selector2/1 -> Divide/1
  Divide/1 -> Discrete Derivative2/1
  PQ_pre/1 -> MATLAB Function1/6(i_pq_pre)
  i abs_pre/1 -> MATLAB Function1/7(i_abs_pre)
  Transport Delay/1 -> Add/2
  Add/1 -> Scope/2, MATLAB Function1/8(u_diff)
  i_inv/1 -> Selector1/1, Selector2/1, T->ControlSampleTime/1(In1), MATLAB Function1/1(i_inv)
  Selector1/1 -> Divide1/1
  Divide1/1 -> Discrete Derivative1/1
  Abs/1 -> Mean/1
  Discrete Derivative2/1 -> Abs/1
  Mean/1 -> MATLAB Function1/4(der)

== system AGI_hydrogen/Battery/VSM1/VSM/MANAGEMENT/Subsystem1/Subsystem1 ==
  In1 : Inport
  In2 : Inport  Port=2
  Enable : EnablePort
  i_pq_pre : Outport
  i_abs_pre : Outport  Port=2
  wires:
  In1/1 -> i_pq_pre/1
  In2/1 -> i_abs_pre/1

== system AGI_hydrogen/Battery/VSM1/VSM/MANAGEMENT/sp_VSM/E(PQ) ==
  E : Inport
  cmd : Inport  Port=2
  sp_PQ : Inport  Port=3
  Abs : Abs  SaturateOnIntegerOverflow=off
  Add : Sum
  Add1 : Sum  Inputs=--
  Add2 : Sum  Inputs=+++
  Bus Selector : BusSelector  OutputSignals=Param.VC.R1,Param.VC.R1t,Param.VC.L1,Param.VC.L1t,Param.VSM.ku
  Bus Selector1 : BusSelector  OutputSignals=Param.VSM.sp_E_comp
  Constant : Constant
  Demux : Demux  Outputs=2
  Display{,1..4} (5 alike) : Display
  Divide : Product  Inputs=/*
  Product : Product
  Product1 : Product
  Real-Imag to Complex : RealImagToComplex
  Real-Imag to Complex1 : RealImagToComplex
  Switch : Switch  Criteria=u2 ~= 0  SaturateOnIntegerOverflow=off  InputSameDT=off
  "cmd " : InportShadow  Port=2
  sp_E : Outport  VectorParamsAs1DForOutWhenUnconnected=off
  wires:
  Add2/1 -> Display3/1, Abs/1
  Abs/1 -> Display4/1, Switch/1
  Product/1 -> Display2/1, Add2/2  "voltage"
  Real-Imag to Complex/1 -> Display1/1, Product/2  "impedance"
  Divide/1 -> Display/1, Product/1  "current"
  Real-Imag to Complex1/1 -> Divide/2
  Demux/2 -> Product1/1, Real-Imag to Complex1/2
  Demux/1 -> Real-Imag to Complex1/1
  sp_PQ/1 -> Demux/1
  E/1 -> Switch/3
  Add1/1 -> Real-Imag to Complex/2
  Add/1 -> Real-Imag to Complex/1
  Bus Selector/4 -> Add1/2  "<L1t>"
  Bus Selector/3 -> Add1/1  "<L1>"
  Bus Selector/2 -> Add/2  "<R1t>"
  Bus Selector/1 -> Add/1  "<R1>"
  cmd/1 -> Bus Selector/1
  Switch/1 -> sp_E/1
  "cmd "/1 -> Bus Selector1/1
  Bus Selector1/1 -> Switch/2  "<sp_E_comp>"
  Bus Selector/5 -> Product1/2  "<ku>"
  Product1/1 -> Add2/3
  Constant/1 -> Divide/1, Add2/1

== system AGI_hydrogen/Battery/VSM1/VSM/MANAGEMENT/sp_VSM/PQ(U) Limit ==
  note: hier muss mit der Leistungsvorgabe multipliziert werden
      | 0.8 U * P0
  sp_PQ : Inport
  enable : Inport  Port=2
  u_out : Inport  Port=3
  Add : Sum
  Constant : Constant
  Dead Zone : DeadZone  LowerValue=0.95  UpperValue=1.05
  Demux : Demux  Outputs=2
  Demux1 : Demux  Outputs=2
  Math Function : Math  Operator=hypot  SignedPower=on
  MinMax : MinMax  Inputs=2
  Mux : Mux  Inputs=2
  Product : Product
  Scope : Scope
  Selector2 : Selector  InputPortWidth=3  IndexOptions=Index vector (dialog)  Indices=[1 2]  OutputSizes=1
  Switch : Switch  Criteria=u2 ~= 0  SaturateOnIntegerOverflow=off  InputSameDT=off
  sp_PQ_limit : Outport  VectorParamsAs1DForOutWhenUnconnected=off
  wires:
  Selector2/1 -> Demux/1
  Demux/1 -> Math Function/1
  Demux/2 -> Math Function/2
  Math Function/1 -> Dead Zone/1
  u_out/1 -> Selector2/1
  sp_PQ/1 -> Switch/3, Demux1/1
  Demux1/2 -> Mux/2
  Demux1/1 -> MinMax/2, Product/2
  MinMax/1 -> Mux/1
  Mux/1 -> Switch/1
  Switch/1 -> Scope/1, sp_PQ_limit/1
  enable/1 -> Switch/2
  Product/1 -> MinMax/1
  Dead Zone/1 -> Add/2
  Add/1 -> Product/1
  Constant/1 -> Add/1

== system AGI_hydrogen/Battery/VSM1/VSM/MANAGEMENT/sp_VSM/RateLimit ==
  PQ : Inport
  Enable : EnablePort
  Compare To Zero : simulink/Logic and Bit Operations/Compare To Zero  relop=>  OutDataTypeStr=boolean
  Constant1 : Constant  Value=Mgn.PQSpRateUp  SampleTime=ControlSampleTime
  Constant2 : Constant  Value=Mgn.PQSpRateDown  SampleTime=ControlSampleTime
  Constant6 : Constant  Value=Mgn.PQSpRateDown  SampleTime=ControlSampleTime
  Constant7 : Constant  Value=Mgn.PQSpRateUp  SampleTime=ControlSampleTime
  Constant8 : Constant  Value=[0 0]  SampleTime=ControlSampleTime
  Logical Operator : Logic  Inputs=1  AllPortsSameDT=off  OutDataTypeStr=boolean
  Mux : Mux  Inputs=2
  Switch : Switch  Criteria=u2 > Threshold  SaturateOnIntegerOverflow=off  InputSameDT=off
  ratelimitspPQ : Subsystem  mask{Ts=ControlSampleTime}
      mask DialogControl ParameterGroupVar Prompt: Rate Limiter
  PQslow : Outport  VectorParamsAs1DForOutWhenUnconnected=off
  wires:
  Logical Operator/1 -> Switch/2
  Mux/1 -> Compare To Zero/1
  Constant2/1 -> Mux/2
  Constant1/1 -> Mux/1
  Compare To Zero/1 -> Logical Operator/1
  Constant7/1 -> ratelimitspPQ/1(rateup)
  Switch/1 -> PQslow/1  "sp_PQ"
  Constant6/1 -> ratelimitspPQ/3(ratedown)
  Constant8/1 -> ratelimitspPQ/4(x0)
  PQ/1 -> ratelimitspPQ/2(x), Switch/1, Switch/3

== system AGI_hydrogen/Battery/VSM1/VSM/CONTROL/VSMOC1/VSMOC/Enabled Subsystem ==
  u_abs : Inport
  Enable : EnablePort
  Out1 : Outport
  wires:
  u_abs/1 -> Out1/1

== system AGI_hydrogen/Battery/VSM1/VSM/CONTROL/VSMOC1/VSMOC/Enabled Subsystem1 ==
  P : Inport
  Enable : EnablePort
  Out1 : Outport
  wires:
  P/1 -> Out1/1

== system AGI_hydrogen/Battery/VSM1/VSM/CONTROL/VSMOC1/VSMOC/FRT Slow Down ==
  U : Inport
  Bias : Bias  Bias=0.2  SaturateOnIntegerOverflow=off
  Complex to Magnitude-Angle : ComplexToMagnitudeAngle
  Demux : Demux  Outputs=2
  Real-Imag to Complex : RealImagToComplex
  Saturation : Saturate  UpperLimit=1  LowerLimit=0
  Terminator : Terminator
  Unit Delay4 : UnitDelay  SampleTime=ControlSampleTime  HasFrameUpgradeWarning=on
  K : Outport  VectorParamsAs1DForOutWhenUnconnected=off
  wires:
  Complex to Magnitude-Angle/1 -> Bias/1
  Demux/2 -> Real-Imag to Complex/2
  Demux/1 -> Real-Imag to Complex/1
  Real-Imag to Complex/1 -> Complex to Magnitude-Angle/1
  U/1 -> Unit Delay4/1
  Complex to Magnitude-Angle/2 -> Terminator/1
  Bias/1 -> Saturation/1
  Saturation/1 -> K/1
  Unit Delay4/1 -> Demux/1

== system AGI_hydrogen/Battery/VSM1/VSM/CONTROL/VSMOC1/VSMOC/Integrator (Angle) ==
  Reset : Inport
  omega : Inport  Port=2
  d_phi0 : Inport  Port=3
  Angle Integrator Reset[SI] : FriedrichLibrary/Discrete Stuff/Angle Integrator Reset[SI]  Ts=ControlSampleTime
  Delay : Delay  DelayLength=1  InitialConditionSource=Input port
      settings: InputPortMap=u0,p4
  Gain3 : Gain  Gain=-1*ControlSampleTime
  Scope : Scope  NumInputPorts=2
  Scope1 : Scope  NumInputPorts=2
  Sum1 : Sum  Inputs=|++
  Sum9 : Sum  Inputs=|+-
  phi : Outport  VectorParamsAs1DForOutWhenUnconnected=off
  wires:
  Gain3/1 -> Sum9/2, Scope/2, Delay/2
  omega/1 -> Gain3/1, Angle Integrator Reset[SI]/2
  Angle Integrator Reset[SI]/1 -> Delay/1, phi/1  "Phi [rad]"
  Reset/1 -> Scope1/1, Angle Integrator Reset[SI]/1
  Sum9/1 -> Sum1/1
  Sum1/1 -> Scope1/2, Angle Integrator Reset[SI]/3
  d_phi0/1 -> Sum9/1
  Delay/1 -> Scope/1, Sum1/2

== system AGI_hydrogen/Battery/VSM1/VSM/CONTROL/VSMOC1/VSMOC/Integrator (Inertia) ==
  dPTa : Inport
  omega0 [pu] : Inport  Port=2
  Enable : EnablePort
  Integrator (inertia) : DiscreteIntegrator  gainval=1  InitialConditionSource=external  InitialCondition=1  SampleTime=ControlSampleTime  ICPrevOutput=DiscIntNeverNeededParam  ICPrevScaledInput=DiscIntNeverNeededParam
  omega [pu] : Outport  VectorParamsAs1DForOutWhenUnconnected=off
  wires:
  omega0 [pu]/1 -> Integrator (inertia)/2
  Integrator (inertia)/1 -> omega [pu]/1  "Omega [pu]"
  dPTa/1 -> Integrator (inertia)/1

== system AGI_hydrogen/Battery/VSM1/VSM/CONTROL/VSMOC1/VSMOC/P Filter Init ==
  Tau : Inport
  dP0 : Inport  Port=2
  Enable : EnablePort  StatesWhenEnabling=reset
  Divide4 : Product  Inputs=*/
  Gain : Gain  Gain=-1
  Integrator1 : DiscreteIntegrator  gainval=1  InitialConditionSource=external  SampleTime=ControlSampleTime  ICPrevOutput=DiscIntNeverNeededParam  ICPrevScaledInput=DiscIntNeverNeededParam
  dP : Outport  VectorParamsAs1DForOutWhenUnconnected=off
  wires:
  dP0/1 -> Integrator1/2
  Gain/1 -> Divide4/1
  Divide4/1 -> Integrator1/1
  Tau/1 -> Divide4/2
  Integrator1/1 -> dP/1, Gain/1

== system AGI_hydrogen/Battery/VSM1/VSM/CONTROL/VSMOC1/VSMOC/Q(U)-PI-Regler ==
  Tau : Inport
  E : Inport  Port=2
  E0 : Inport  Port=3
  Enable : EnablePort  StatesWhenEnabling=reset
  Divide2 : Product  Inputs=*/
  Integrator : DiscreteIntegrator  gainval=1  InitialConditionSource=external  InitialCondition=0.9  SampleTime=ControlSampleTime  ICPrevOutput=DiscIntNeverNeededParam  ICPrevScaledInput=DiscIntNeverNeededParam
  Sum1 : Sum  Inputs=|+-
  E_fil : Outport  VectorParamsAs1DForOutWhenUnconnected=off
  wires:
  E0/1 -> Integrator/2
  Divide2/1 -> Integrator/1
  E/1 -> Sum1/1
  Tau/1 -> Divide2/2
  Integrator/1 -> Sum1/2, E_fil/1  "E [pu]"
  Sum1/1 -> Divide2/1

== system AGI_hydrogen/Battery/VSM1/VSM/CONTROL/VSMOC1/VSMOC/Subsystem ==
  first_run : Inport
  u_dq : Inport  Port=2
  u_dq_pll : Inport  Port=3
  phi_pll : Inport  Port=4
  Enable : EnablePort
  Complex to Magnitude-Angle : ComplexToMagnitudeAngle
  Demux : Demux  Outputs=2
  Real-Imag to Complex : RealImagToComplex
  Switch : Switch  Criteria=u2 > Threshold  SaturateOnIntegerOverflow=off  InputSameDT=off
  Switch1 : Switch  Criteria=u2 ~= 0  SaturateOnIntegerOverflow=off  InputSameDT=off
  "first_run " : InportShadow
  u_abs : Outport  InitialOutput=1  VectorParamsAs1DForOutWhenUnconnected=off
  u_ang : Outport  Port=2  InitialOutput=0  VectorParamsAs1DForOutWhenUnconnected=off
  wires:
  Switch/1 -> u_ang/1
  phi_pll/1 -> Switch/1
  Real-Imag to Complex/1 -> Complex to Magnitude-Angle/1
  Demux/1 -> Real-Imag to Complex/1
  Demux/2 -> Real-Imag to Complex/2
  Complex to Magnitude-Angle/1 -> u_abs/1
  Switch1/1 -> Demux/1
  first_run/1 -> Switch1/2
  u_dq/1 -> Switch1/3
  u_dq_pll/1 -> Switch1/1
  "first_run "/1 -> Switch/2
  Complex to Magnitude-Angle/2 -> Switch/3

== system AGI_hydrogen/Battery/VSM1/VSM/MANAGEMENT/Subsystem1/Subsystem/T->ControlSampleTime ==
  In1 : Inport
  Discrete Derivative : simulink/Discrete/Discrete Derivative  gainval=1.0  ICPrevScaledInput=0.0  OutMin=[]  OutMax=[]  OutDataType=fixdt(1, 16)  OutScaling=2^-10  DoSatur=off
  Out1 : Outport
  wires:
  Discrete Derivative/1 -> Out1/1
  In1/1 -> Discrete Derivative/1
